simulink model "AVR_H_2_"  (R2022a)
settings: Solver=VariableStepAuto  StartTime=0.0  StopTime=180  RelTol=1e-3
libraries: simulink x1
settings Model: Creator=asus  LastModifiedBy=asus

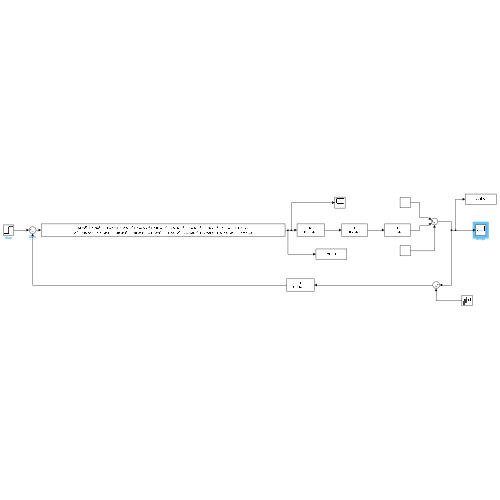
[thumbnail: Simulink's stored preview of the top-level diagram]
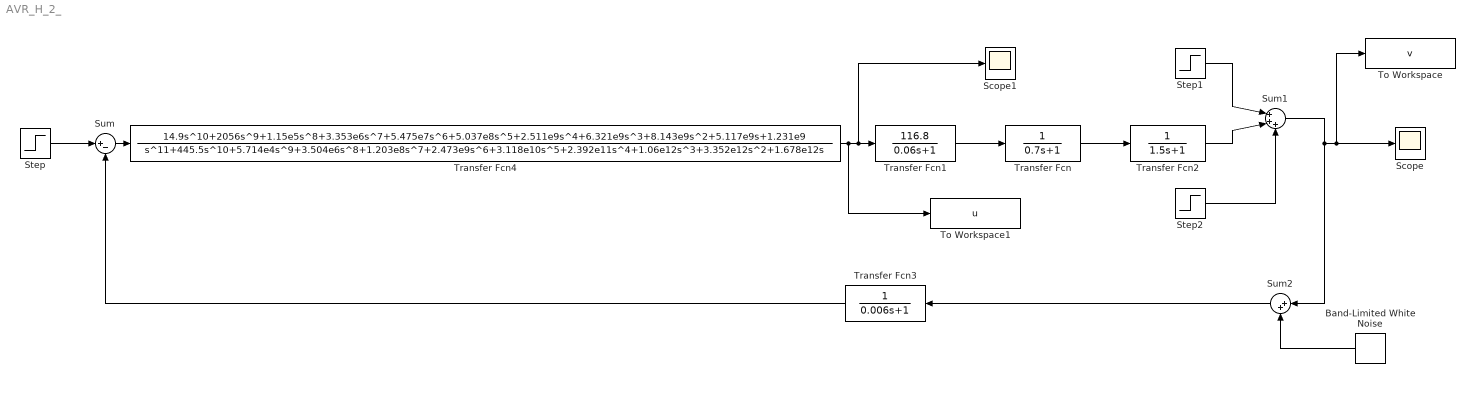
== system AVR_H_2_ ==
  Band-Limited White Noise : simulink/Sources/Band-Limited White Noise  Cov=[0]  Ts=0.1  seed=[23341]
  Scope : Scope
  Scope1 : Scope
  Step : Step  Time=0  SampleTime=0
  Step1 : Step  Time=60  SampleTime=0
  Step2 : Step  Time=120  After=-1  SampleTime=0
  Sum : Sum  Inputs=|+-
  Sum1 : Sum  Inputs=|+++
  Sum2 : Sum  Inputs=|++
  To Workspace : ToWorkspace  VariableName=v  SaveFormat=Timeseries  SampleTime=-1
  To Workspace1 : ToWorkspace  VariableName=u  SaveFormat=Timeseries  SampleTime=-1
  Transfer Fcn : TransferFcn  Denominator=[0.7 1]
  Transfer Fcn1 : TransferFcn  Numerator=[116.8]  Denominator=[0.06 1]
  Transfer Fcn2 : TransferFcn  Denominator=[1.5 1]
  Transfer Fcn3 : TransferFcn  Denominator=[0.006 1]
  Transfer Fcn4 : TransferFcn  Numerator=[14.9 2056 1.15e5 3.353e6 5.475e7 5.037e8 2.511e9 6.321e9 8.143e9 5.117e9 1.231e9]  Denominator=[1 445.5 5.714e4 3.504e6 1.203e8 2.473e9 3.118e10 2.392e11 1.06e12 3.352e12 1.678e12 0]
  wires:
  Transfer Fcn4/1 -> To Workspace1/1, Scope1/1, Transfer Fcn1/1
  Sum1/1 -> Sum2/1, To Workspace/1, Scope/1
  Step2/1 -> Sum1/3
  Transfer Fcn/1 -> Transfer Fcn2/1
  Step/1 -> Sum/1
  Transfer Fcn2/1 -> Sum1/2
  Transfer Fcn3/1 -> Sum/2
  Sum2/1 -> Transfer Fcn3/1
  Step1/1 -> Sum1/1
  Band-Limited White Noise/1 -> Sum2/2
  Transfer Fcn1/1 -> Transfer Fcn/1
  Sum/1 -> Transfer Fcn4/1
